simulink library "CH_Library"  (R2021a)
settings: Solver=VariableStepAuto  StartTime=0.0  StopTime=10.0  RelTol=1e-3
undefined symbols (not defined in the file or in its folder): Connection1, connection1, Connection2, connection2, Connection3, connection3, Connection4, connection4, Connection5, connection5, Connection6, connection6, Connection7, Connection8, FeetContact, HandContact, LeftArm, LeftFoot, params, RightArm, RightFoot, X, Y, Z
libraries: sm_lib x169, nesl_utility x40, $bdroot x16, sm_humanoid_walker_lib x13, fl_lib x10, simulink x7, ee_lib x3, simulink_extras x1
(part 2 of 5)

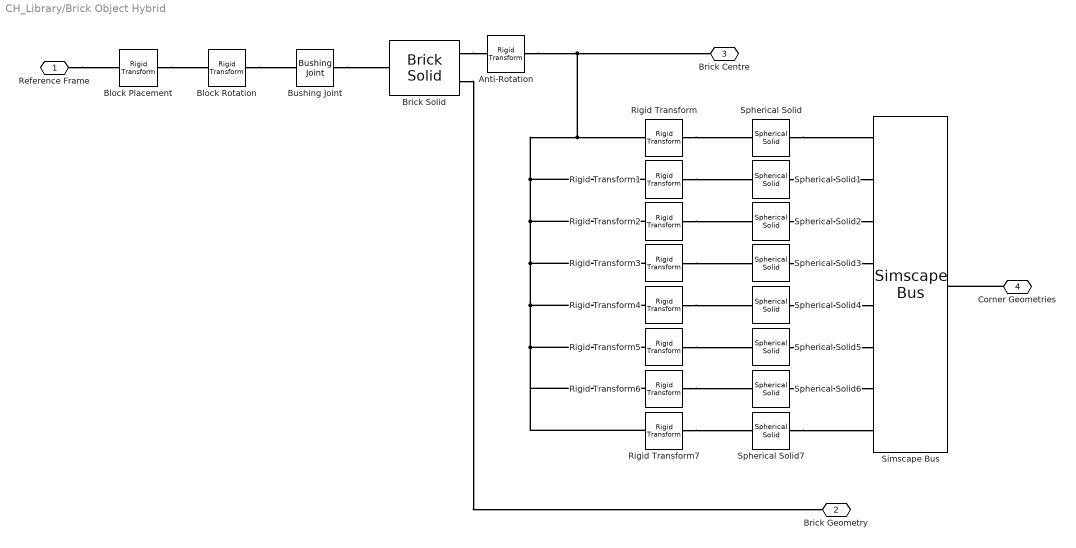
== system CH_Library/Brick Object Hybrid ==
  Anti-Rotation : sm_lib/Frames and Transforms/Rigid Transform  TranslationMethod=None  TranslationStandardOffset=0  TranslationLengthUnit=m  TranslationStandardAxis=+Z  TranslationCartesianOffset=[0 0 0]  TranslationROffset=0  TranslationROffsetUnits=m  TranslationZOffset=0  TranslationZOffsetUnits=m  TranslationThetaOffset=0  TranslationThetaOffsetUnits=deg  RotationMethod=RotationSequence  RotationAngleUnits=deg  RotationStandardAxis=+Z  RotationAngle=0.0  RotationArbitraryAxis=[0 0 1]  FollAlignAxisA=+X  BaseAlignAxisA=+Y  FollAlignAxisB=+Y  BaseAlignAxisB=+Z  RotationSequenceAxes=BaseAxes  RotationSequence=XYZ  RotationSequenceAngles=[-XRot -YRot -ZRot]  RotationSequenceAnglesUnits=deg  RotationMatrix=[1 0 0; 0 1 0; 0 0 1]
  Block Placement : sm_lib/Frames and Transforms/Rigid Transform  TranslationMethod=Cartesian  TranslationStandardOffset=0  TranslationLengthUnit=m  TranslationStandardAxis=+Z  TranslationCartesianOffset=[XDis YDis ZDis]  TranslationROffset=0  TranslationROffsetUnits=m  TranslationZOffset=0  TranslationZOffsetUnits=m  TranslationThetaOffset=0  TranslationThetaOffsetUnits=deg  RotationMethod=None  RotationAngleUnits=deg  RotationStandardAxis=+Z  RotationAngle=0.0  RotationArbitraryAxis=[0 0 1]  FollAlignAxisA=+X  BaseAlignAxisA=+Y  FollAlignAxisB=+Y  BaseAlignAxisB=+Z  RotationSequenceAxes=FollowerAxes  RotationSequence=XYX  RotationSequenceAngles=[0 0 0]  RotationSequenceAnglesUnits=deg  RotationMatrix=[1 0 0; 0 1 0; 0 0 1]
  Block Rotation : sm_lib/Frames and Transforms/Rigid Transform  TranslationMethod=None  TranslationStandardOffset=0  TranslationLengthUnit=m  TranslationStandardAxis=+Z  TranslationCartesianOffset=[0 0 0]  TranslationROffset=0  TranslationROffsetUnits=m  TranslationZOffset=0  TranslationZOffsetUnits=m  TranslationThetaOffset=0  TranslationThetaOffsetUnits=deg  RotationMethod=RotationSequence  RotationAngleUnits=deg  RotationStandardAxis=+Z  RotationAngle=0.0  RotationArbitraryAxis=[0 0 1]  FollAlignAxisA=+X  BaseAlignAxisA=+Y  FollAlignAxisB=+Y  BaseAlignAxisB=+Z  RotationSequenceAxes=BaseAxes  RotationSequence=XYZ  RotationSequenceAngles=[XRot YRot ZRot]  RotationSequenceAnglesUnits=deg  RotationMatrix=[1 0 0; 0 1 0; 0 0 1]
  Brick Solid : sm_lib/Body Elements/Brick Solid  GraphicAmbientColor=[0.15 0.15 0.15 1.0]  BasedOnType=Density  BrickDimensions=[BW BDep BH]  BrickDimensionUnits=m  CenterOfMass=[0 0 0]  CenterOfMassUnits=m  GraphicDiffuseColor=[BlockRed BlockGreen BlockBlue]  Density=BDen  DensityUnits=kg/m^3  DoExposeReferenceFrame=on  GraphicEmissiveColor=[0.0 0.0 0.0 1.0]  ExportEntireGeometry=on  SerializedFrames=<Frames><Frame><Id>Frame1</Id><Value><Name>Block Centre</Name><Origin><Source>ReferenceFrame</Source><FeatureName></FeatureName></Origin><PrimaryAxis><DefinedDirection>+Z</DefinedDirection><Source>ReferenceFrame</Source><SourceDirection>+Z</SourceDirection><FeatureName></FeatureName></PrimaryAxis><SecondaryAxis><DefinedDirection>+X</DefinedDirection><Source>ReferenceFrame</Source><SourceDirection>+X</SourceDirection><FeatureName></FeatureName></SecondaryAxis></Value></Frame></Frames>  MarkerShape=Sphere  MarkerSize=10  GraphicType=FromGeometry  InertiaType=CalculateFromGeometry  Mass=1  MassUnits=kg  MomentsOfInertia=[1 1 1]  MomentsOfInertiaUnits=kg*m^2  GraphicOpacity=BlockOpac  ProductsOfInertia=[0 0 0]  ProductsOfInertiaUnits=kg*m^2  GraphicShininess=75  GraphicSpecularColor=[0.5 0.5 0.5 1.0]  GraphicVisPropType=SimpleVisualProperties
  Bushing Joint : sm_lib/Joints/Bushing Joint  JointMode=Normal  SenseConstraintForce=off  SenseConstraintForceX=off  SenseConstraintForceY=off  SenseConstraintForceZ=off  SenseConstraintTorque=off  SenseConstraintTorqueX=off  SenseConstraintTorqueY=off  SenseConstraintTorqueZ=off  SenseTotalForce=off  SenseTotalForceX=off  SenseTotalForceY=off  SenseTotalForceZ=off  SenseTotalTorque=off  SenseTotalTorqueX=off  SenseTotalTorqueY=off  SenseTotalTorqueZ=off  CompositeWrenchDir=FollowerOnBase  CompositeWrenchFrame=BaseFrame  PxEquilibriumPosition=0  PxEquilibriumPositionUnits=m  PxSpringStiffness=0  PxSpringStiffnessUnits=N/m  PxDampingCoefficient=0  PxDampingCoefficientUnits=N/(m/s)  PxTorqueActuationMode=NoTorque  PxMotionActuationMode=ComputedMotion  PxSensePosition=off  PxSenseVelocity=off  PxSenseAcceleration=off  PxSenseTorqueForce=off  PxSenseLowerLimitTorqueForce=off  PxSenseUpperLimitTorqueForce=off  PxLowerLimitSpecify=off  PxLowerLimitBound=-1  PxLowerLimitBoundUnits=m  PxLowerLimitStiffness=1e6  PxLowerLimitStiffnessUnits=N/m  PxLowerLimitDamping=1e3  PxLowerLimitDampingUnits=N/(m/s)  PxLowerLimitTransitionRegionWidth=1e-4  PxLowerLimitTransitionRegionWidthUnits=m  PxUpperLimitSpecify=off  PxUpperLimitBound=1  PxUpperLimitBoundUnits=m  PxUpperLimitStiffness=1e6  PxUpperLimitStiffnessUnits=N/m  PxUpperLimitDamping=1e3  PxUpperLimitDampingUnits=N/(m/s)  PxUpperLimitTransitionRegionWidth=1e-4  PxUpperLimitTransitionRegionWidthUnits=m  PxPositionTargetSpecify=off  PxPositionTargetPriority=High  PxPositionTargetValue=0  PxPositionTargetValueUnits=m  PxVelocityTargetSpecify=off  PxVelocityTargetPriority=High  PxVelocityTargetValue=0  PxVelocityTargetValueUnits=m/s  PyEquilibriumPosition=0  PyEquilibriumPositionUnits=m  PySpringStiffness=0  PySpringStiffnessUnits=N/m  PyDampingCoefficient=0  PyDampingCoefficientUnits=N/(m/s)  PyTorqueActuationMode=NoTorque  PyMotionActuationMode=ComputedMotion  PySensePosition=off  PySenseVelocity=off  PySenseAcceleration=off  PySenseTorqueForce=off  PySenseLowerLimitTorqueForce=off  PySenseUpperLimitTorqueForce=off  PyLowerLimitSpecify=off  PyLowerLimitBound=-1  PyLowerLimitBoundUnits=m  PyLowerLimitStiffness=1e6  PyLowerLimitStiffnessUnits=N/m  PyLowerLimitDamping=1e3  PyLowerLimitDampingUnits=N/(m/s)  PyLowerLimitTransitionRegionWidth=1e-4  PyLowerLimitTransitionRegionWidthUnits=m  PyUpperLimitSpecify=off  PyUpperLimitBound=1  PyUpperLimitBoundUnits=m  PyUpperLimitStiffness=1e6  PyUpperLimitStiffnessUnits=N/m  PyUpperLimitDamping=1e3  PyUpperLimitDampingUnits=N/(m/s)  PyUpperLimitTransitionRegionWidth=1e-4  PyUpperLimitTransitionRegionWidthUnits=m  PyPositionTargetSpecify=off  PyPositionTargetPriority=High  PyPositionTargetValue=0  PyPositionTargetValueUnits=m  PyVelocityTargetSpecify=off  PyVelocityTargetPriority=High  PyVelocityTargetValue=0  PyVelocityTargetValueUnits=m/s  PzEquilibriumPosition=0  PzEquilibriumPositionUnits=m  PzSpringStiffness=0  PzSpringStiffnessUnits=N/m  PzDampingCoefficient=0  PzDampingCoefficientUnits=N/(m/s)  PzTorqueActuationMode=NoTorque  PzMotionActuationMode=ComputedMotion  PzSensePosition=off  PzSenseVelocity=off  PzSenseAcceleration=off  PzSenseTorqueForce=off  PzSenseLowerLimitTorqueForce=off  PzSenseUpperLimitTorqueForce=off  PzLowerLimitSpecify=off  PzLowerLimitBound=-1  PzLowerLimitBoundUnits=m  PzLowerLimitStiffness=1e6  PzLowerLimitStiffnessUnits=N/m  PzLowerLimitDamping=1e3  PzLowerLimitDampingUnits=N/(m/s)  PzLowerLimitTransitionRegionWidth=1e-4  PzLowerLimitTransitionRegionWidthUnits=m  PzUpperLimitSpecify=off  PzUpperLimitBound=1  PzUpperLimitBoundUnits=m  PzUpperLimitStiffness=1e6  PzUpperLimitStiffnessUnits=N/m  PzUpperLimitDamping=1e3  PzUpperLimitDampingUnits=N/(m/s)  PzUpperLimitTransitionRegionWidth=1e-4  PzUpperLimitTransitionRegionWidthUnits=m  PzPositionTargetSpecify=off  PzPositionTargetPriority=High  PzPositionTargetValue=0  PzPositionTargetValueUnits=m  PzVelocityTargetSpecify=off  PzVelocityTargetPriority=High  PzVelocityTargetValue=0  PzVelocityTargetValueUnits=m/s  RxEquilibriumPosition=0  RxEquilibriumPositionUnits=deg  RxSpringStiffness=0  RxSpringStiffnessUnits=N*m/deg  RxDampingCoefficient=0  RxDampingCoefficientUnits=N*m/(deg/s)  RxTorqueActuationMode=NoTorque  RxMotionActuationMode=ComputedMotion  RxSensePosition=off  RxSenseVelocity=off  RxSenseAcceleration=off  RxSenseTorqueForce=off  RxSenseLowerLimitTorqueForce=off  RxSenseUpperLimitTorqueForce=off  RxLowerLimitSpecify=off  RxLowerLimitBound=-90  RxLowerLimitBoundUnits=deg  RxLowerLimitStiffness=1e4  RxLowerLimitStiffnessUnits=N*m/deg  RxLowerLimitDamping=10  RxLowerLimitDampingUnits=N*m/(deg/s)  RxLowerLimitTransitionRegionWidth=0.1  RxLowerLimitTransitionRegionWidthUnits=deg  RxUpperLimitSpecify=off  RxUpperLimitBound=90  RxUpperLimitBoundUnits=deg  RxUpperLimitStiffness=1e4  RxUpperLimitStiffnessUnits=N*m/deg  RxUpperLimitDamping=10  RxUpperLimitDampingUnits=N*m/(deg/s)  RxUpperLimitTransitionRegionWidth=0.1  RxUpperLimitTransitionRegionWidthUnits=deg  RxPositionTargetSpecify=off  RxPositionTargetPriority=High  RxPositionTargetValue=0  RxPositionTargetValueUnits=deg  RxVelocityTargetSpecify=off  RxVelocityTargetPriority=High  RxVelocityTargetValue=0  RxVelocityTargetValueUnits=deg/s  RyEquilibriumPosition=0  RyEquilibriumPositionUnits=deg  RySpringStiffness=0  RySpringStiffnessUnits=N*m/deg  RyDampingCoefficient=0  RyDampingCoefficientUnits=N*m/(deg/s)  RyTorqueActuationMode=NoTorque  RyMotionActuationMode=ComputedMotion  RySensePosition=off  RySenseVelocity=off  RySenseAcceleration=off  RySenseTorqueForce=off  RySenseLowerLimitTorqueForce=off  RySenseUpperLimitTorqueForce=off  RyLowerLimitSpecify=off  RyLowerLimitBound=-90  RyLowerLimitBoundUnits=deg  RyLowerLimitStiffness=1e4  RyLowerLimitStiffnessUnits=N*m/deg  RyLowerLimitDamping=10  RyLowerLimitDampingUnits=N*m/(deg/s)  RyLowerLimitTransitionRegionWidth=0.1  RyLowerLimitTransitionRegionWidthUnits=deg  RyUpperLimitSpecify=off  RyUpperLimitBound=90  RyUpperLimitBoundUnits=deg  RyUpperLimitStiffness=1e4  RyUpperLimitStiffnessUnits=N*m/deg  RyUpperLimitDamping=10  RyUpperLimitDampingUnits=N*m/(deg/s)  RyUpperLimitTransitionRegionWidth=0.1  RyUpperLimitTransitionRegionWidthUnits=deg  RyPositionTargetSpecify=off  RyPositionTargetPriority=High  RyPositionTargetValue=0  RyPositionTargetValueUnits=deg  RyVelocityTargetSpecify=off  RyVelocityTargetPriority=High  RyVelocityTargetValue=0  RyVelocityTargetValueUnits=deg/s  RzEquilibriumPosition=0  RzEquilibriumPositionUnits=deg  RzSpringStiffness=0  RzSpringStiffnessUnits=N*m/deg  RzDampingCoefficient=0  RzDampingCoefficientUnits=N*m/(deg/s)  RzTorqueActuationMode=NoTorque  RzMotionActuationMode=ComputedMotion  RzSensePosition=off  RzSenseVelocity=off  RzSenseAcceleration=off  RzSenseTorqueForce=off  RzSenseLowerLimitTorqueForce=off  RzSenseUpperLimitTorqueForce=off  RzLowerLimitSpecify=off  RzLowerLimitBound=-90  RzLowerLimitBoundUnits=deg  RzLowerLimitStiffness=1e4  RzLowerLimitStiffnessUnits=N*m/deg  RzLowerLimitDamping=10  RzLowerLimitDampingUnits=N*m/(deg/s)  RzLowerLimitTransitionRegionWidth=0.1  RzLowerLimitTransitionRegionWidthUnits=deg  RzUpperLimitSpecify=off  RzUpperLimitBound=90  RzUpperLimitBoundUnits=deg  RzUpperLimitStiffness=1e4  RzUpperLimitStiffnessUnits=N*m/deg  RzUpperLimitDamping=10  RzUpperLimitDampingUnits=N*m/(deg/s)  RzUpperLimitTransitionRegionWidth=0.1  RzUpperLimitTransitionRegionWidthUnits=deg  RzPositionTargetSpecify=off  RzPositionTargetPriority=High  RzPositionTargetValue=0  RzPositionTargetValueUnits=deg  RzVelocityTargetSpecify=off  RzVelocityTargetPriority=High  RzVelocityTargetValue=0  RzVelocityTargetValueUnits=deg/s
  Rigid Transform : sm_lib/Frames and Transforms/Rigid Transform  TranslationMethod=Cartesian  TranslationStandardOffset=0  TranslationLengthUnit=m  TranslationStandardAxis=+Z  TranslationCartesianOffset=[BW BH BDep]/2  TranslationROffset=0  TranslationROffsetUnits=m  TranslationZOffset=0  TranslationZOffsetUnits=m  TranslationThetaOffset=0  TranslationThetaOffsetUnits=deg  RotationMethod=None  RotationAngleUnits=deg  RotationStandardAxis=+Z  RotationAngle=0.0  RotationArbitraryAxis=[0 0 1]  FollAlignAxisA=+X  BaseAlignAxisA=+Y  FollAlignAxisB=+Y  BaseAlignAxisB=+Z  RotationSequenceAxes=FollowerAxes  RotationSequence=XYX  RotationSequenceAngles=[0 0 0]  RotationSequenceAnglesUnits=deg  RotationMatrix=[1 0 0; 0 1 0; 0 0 1]
  Rigid Transform1 : sm_lib/Frames and Transforms/Rigid Transform  TranslationMethod=Cartesian  TranslationStandardOffset=0  TranslationLengthUnit=m  TranslationStandardAxis=+Z  TranslationCartesianOffset=[BW BH -BDep]/2  TranslationROffset=0  TranslationROffsetUnits=m  TranslationZOffset=0  TranslationZOffsetUnits=m  TranslationThetaOffset=0  TranslationThetaOffsetUnits=deg  RotationMethod=None  RotationAngleUnits=deg  RotationStandardAxis=+Z  RotationAngle=0.0  RotationArbitraryAxis=[0 0 1]  FollAlignAxisA=+X  BaseAlignAxisA=+Y  FollAlignAxisB=+Y  BaseAlignAxisB=+Z  RotationSequenceAxes=FollowerAxes  RotationSequence=XYX  RotationSequenceAngles=[0 0 0]  RotationSequenceAnglesUnits=deg  RotationMatrix=[1 0 0; 0 1 0; 0 0 1]
  Rigid Transform2 : sm_lib/Frames and Transforms/Rigid Transform  TranslationMethod=Cartesian  TranslationStandardOffset=0  TranslationLengthUnit=m  TranslationStandardAxis=+Z  TranslationCartesianOffset=[BW -BH BDep]/2  TranslationROffset=0  TranslationROffsetUnits=m  TranslationZOffset=0  TranslationZOffsetUnits=m  TranslationThetaOffset=0  TranslationThetaOffsetUnits=deg  RotationMethod=None  RotationAngleUnits=deg  RotationStandardAxis=+Z  RotationAngle=0.0  RotationArbitraryAxis=[0 0 1]  FollAlignAxisA=+X  BaseAlignAxisA=+Y  FollAlignAxisB=+Y  BaseAlignAxisB=+Z  RotationSequenceAxes=FollowerAxes  RotationSequence=XYX  RotationSequenceAngles=[0 0 0]  RotationSequenceAnglesUnits=deg  RotationMatrix=[1 0 0; 0 1 0; 0 0 1]
  Rigid Transform3 : sm_lib/Frames and Transforms/Rigid Transform  TranslationMethod=Cartesian  TranslationStandardOffset=0  TranslationLengthUnit=m  TranslationStandardAxis=+Z  TranslationCartesianOffset=[BW -BH -BDep]/2  TranslationROffset=0  TranslationROffsetUnits=m  TranslationZOffset=0  TranslationZOffsetUnits=m  TranslationThetaOffset=0  TranslationThetaOffsetUnits=deg  RotationMethod=None  RotationAngleUnits=deg  RotationStandardAxis=+Z  RotationAngle=0.0  RotationArbitraryAxis=[0 0 1]  FollAlignAxisA=+X  BaseAlignAxisA=+Y  FollAlignAxisB=+Y  BaseAlignAxisB=+Z  RotationSequenceAxes=FollowerAxes  RotationSequence=XYX  RotationSequenceAngles=[0 0 0]  RotationSequenceAnglesUnits=deg  RotationMatrix=[1 0 0; 0 1 0; 0 0 1]
  Rigid Transform4 : sm_lib/Frames and Transforms/Rigid Transform  TranslationMethod=Cartesian  TranslationStandardOffset=0  TranslationLengthUnit=m  TranslationStandardAxis=+Z  TranslationCartesianOffset=[-BW BH BDep]/2  TranslationROffset=0  TranslationROffsetUnits=m  TranslationZOffset=0  TranslationZOffsetUnits=m  TranslationThetaOffset=0  TranslationThetaOffsetUnits=deg  RotationMethod=None  RotationAngleUnits=deg  RotationStandardAxis=+Z  RotationAngle=0.0  RotationArbitraryAxis=[0 0 1]  FollAlignAxisA=+X  BaseAlignAxisA=+Y  FollAlignAxisB=+Y  BaseAlignAxisB=+Z  RotationSequenceAxes=FollowerAxes  RotationSequence=XYX  RotationSequenceAngles=[0 0 0]  RotationSequenceAnglesUnits=deg  RotationMatrix=[1 0 0; 0 1 0; 0 0 1]
  Rigid Transform5 : sm_lib/Frames and Transforms/Rigid Transform  TranslationMethod=Cartesian  TranslationStandardOffset=0  TranslationLengthUnit=m  TranslationStandardAxis=+Z  TranslationCartesianOffset=[-BW BH -BDep]/2  TranslationROffset=0  TranslationROffsetUnits=m  TranslationZOffset=0  TranslationZOffsetUnits=m  TranslationThetaOffset=0  TranslationThetaOffsetUnits=deg  RotationMethod=None  RotationAngleUnits=deg  RotationStandardAxis=+Z  RotationAngle=0.0  RotationArbitraryAxis=[0 0 1]  FollAlignAxisA=+X  BaseAlignAxisA=+Y  FollAlignAxisB=+Y  BaseAlignAxisB=+Z  RotationSequenceAxes=FollowerAxes  RotationSequence=XYX  RotationSequenceAngles=[0 0 0]  RotationSequenceAnglesUnits=deg  RotationMatrix=[1 0 0; 0 1 0; 0 0 1]
  Rigid Transform6 : sm_lib/Frames and Transforms/Rigid Transform  TranslationMethod=Cartesian  TranslationStandardOffset=0  TranslationLengthUnit=m  TranslationStandardAxis=+Z  TranslationCartesianOffset=[-BW -BH BDep]/2  TranslationROffset=0  TranslationROffsetUnits=m  TranslationZOffset=0  TranslationZOffsetUnits=m  TranslationThetaOffset=0  TranslationThetaOffsetUnits=deg  RotationMethod=None  RotationAngleUnits=deg  RotationStandardAxis=+Z  RotationAngle=0.0  RotationArbitraryAxis=[0 0 1]  FollAlignAxisA=+X  BaseAlignAxisA=+Y  FollAlignAxisB=+Y  BaseAlignAxisB=+Z  RotationSequenceAxes=FollowerAxes  RotationSequence=XYX  RotationSequenceAngles=[0 0 0]  RotationSequenceAnglesUnits=deg  RotationMatrix=[1 0 0; 0 1 0; 0 0 1]
  Rigid Transform7 : sm_lib/Frames and Transforms/Rigid Transform  TranslationMethod=Cartesian  TranslationStandardOffset=0  TranslationLengthUnit=m  TranslationStandardAxis=+Z  TranslationCartesianOffset=[-BW -BH -BDep]/2  TranslationROffset=0  TranslationROffsetUnits=m  TranslationZOffset=0  TranslationZOffsetUnits=m  TranslationThetaOffset=0  TranslationThetaOffsetUnits=deg  RotationMethod=None  RotationAngleUnits=deg  RotationStandardAxis=+Z  RotationAngle=0.0  RotationArbitraryAxis=[0 0 1]  FollAlignAxisA=+X  BaseAlignAxisA=+Y  FollAlignAxisB=+Y  BaseAlignAxisB=+Z  RotationSequenceAxes=FollowerAxes  RotationSequence=XYX  RotationSequenceAngles=[0 0 0]  RotationSequenceAnglesUnits=deg  RotationMatrix=[1 0 0; 0 1 0; 0 0 1]
  Simscape Bus : SimscapeBus  HierarchyStrings=Connection1;Connection2;Connection3;Connection4;Connection5;Connection6;Connection7;Connection8
  Spherical Solid{,1..7} (8 alike) : sm_lib/Body Elements/Spherical Solid  GraphicAmbientColor=[0.15 0.15 0.15 1.0]  BasedOnType=Density  CenterOfMass=[0 0 0]  CenterOfMassUnits=m  GraphicDiffuseColor=[0.5 0.5 0.5]  Density=0.01  DensityUnits=kg/m^3  DoExposeReferenceFrame=on  GraphicEmissiveColor=[0.0 0.0 0.0 1.0]  ExportEntireGeometry=on  SerializedExposedGeometries=<ExposedGeometries><ExposedGeometry><RawGeometryId>entire</RawGeometryId><ExposedGeometryId>G</ExposedGeometryId></ExposedGeometry></ExposedGeometries>  SerializedFrames=<Frames/>  MarkerShape=Sphere  MarkerSize=10  GraphicType=FromGeometry  InertiaType=CalculateFromGeometry  Mass=1  MassUnits=kg  MomentsOfInertia=[1 1 1]  MomentsOfInertiaUnits=kg*m^2  GraphicOpacity=0  ProductsOfInertia=[0 0 0]  ProductsOfInertiaUnits=kg*m^2  GraphicShininess=75  GraphicSpecularColor=[0.5 0.5 0.5 1.0]  SphereRadius=0.1  SphereRadiusUnits=m  GraphicVisPropType=SimpleVisualProperties
  Reference Frame : PMIOPort  Side=Left
  Brick Geometry : PMIOPort  Port=2  Side=Right
  Brick Centre : PMIOPort  Port=3  Side=Right
  Corner Geometries : PMIOPort  Port=4  Side=Right
  connections:
  Bushing Joint/RConn1 -- Brick Solid/RConn1
  Reference Frame/RConn1 -- Block Placement/LConn1
  Block Placement/RConn1 -- Block Rotation/LConn1
  Block Rotation/RConn1 -- Bushing Joint/LConn1
  Brick Solid/LConn1 -- Anti-Rotation/LConn1
  Rigid Transform3/LConn1 -- Rigid Transform/LConn1 -- Brick Centre/RConn1 -- Anti-Rotation/RConn1 -- Rigid Transform1/LConn1 -- Rigid Transform2/LConn1 -- Rigid Transform4/LConn1 -- Rigid Transform5/LConn1 -- Rigid Transform6/LConn1 -- Rigid Transform7/LConn1
  Brick Solid/LConn2 -- Brick Geometry/RConn1
  Spherical Solid4/LConn1 -- Simscape Bus/LConn5
  Rigid Transform6/RConn1 -- Spherical Solid6/RConn1
  Spherical Solid6/LConn1 -- Simscape Bus/LConn7
  Spherical Solid2/LConn1 -- Simscape Bus/LConn3
  Spherical Solid1/LConn1 -- Simscape Bus/LConn2
  Spherical Solid/LConn1 -- Simscape Bus/LConn1
  Spherical Solid3/LConn1 -- Simscape Bus/LConn4
  Rigid Transform5/RConn1 -- Spherical Solid5/RConn1
  Rigid Transform/RConn1 -- Spherical Solid/RConn1
  Rigid Transform1/RConn1 -- Spherical Solid1/RConn1
  Rigid Transform4/RConn1 -- Spherical Solid4/RConn1
  Spherical Solid7/LConn1 -- Simscape Bus/LConn8
  Spherical Solid5/LConn1 -- Simscape Bus/LConn6
  Rigid Transform7/RConn1 -- Spherical Solid7/RConn1
  Rigid Transform2/RConn1 -- Spherical Solid2/RConn1
  Corner Geometries/RConn1 -- Simscape Bus/RConn1
  Rigid Transform3/RConn1 -- Spherical Solid3/RConn1

== system CH_Library/Calculate Power ==
  Joint Sensing : Inport
  Joint Torques : Inport  Port=2
  Bus Selector1 : BusSelector  OutputSignals=LegSense.RightLegSense.RHS.rhThetaDot,LegSense.RightLegSense.RKS.rkThetaDot,LegSense.RightLegSense.RAS.raThetaDot,LegSense.LeftLegSense.LHS.lhThetaDot,LegSense.LeftLegSense.LKS.lkThetaDot,LegSense.LeftLegSense.LAS.laThetaDot,ArmSense.LeftArmSense.LWS.lwThetaDot,ArmSense.LeftArmSense.LES.leThetaDot,ArmSense.LeftArmSense.LSSS.lssThetaDot,ArmSense.LeftArmSense.LSFS.lsfThetaDot,ArmSense.RightArmSense.RWS.rwThetaDot,ArmSense.RightArmSense.RES.reThetaDot,ArmSense.RightArmSense.RSSS.rssThetaDot,ArmSense.RightArmSense.RSFS.rsfThetaDot
  Mux : Mux  Inputs=14
  Product : Product
  Sum of Elements : Sum  Inputs=+
  Unit Delay : UnitDelay  SampleTime=-1  HasFrameUpgradeWarning=on
  Total Power : Outport
  wires:
  Bus Selector1/7 -> Mux/7  "<lwThetaDot>"
  Bus Selector1/8 -> Mux/8  "<leThetaDot>"
  Bus Selector1/9 -> Mux/9  "<lssThetaDot>"
  Bus Selector1/10 -> Mux/10  "<lsfThetaDot>"
  Bus Selector1/11 -> Mux/11  "<rwThetaDot>"
  Bus Selector1/12 -> Mux/12  "<reThetaDot>"
  Bus Selector1/13 -> Mux/13  "<rssThetaDot>"
  Bus Selector1/14 -> Mux/14  "<rsfThetaDot>"
  Product/1 -> Sum of Elements/1
  Joint Sensing/1 -> Bus Selector1/1
  Mux/1 -> Product/1
  Joint Torques/1 -> Product/2
  Sum of Elements/1 -> Unit Delay/1
  Bus Selector1/1 -> Mux/1  "<rhThetaDot>"
  Bus Selector1/2 -> Mux/2  "<rkThetaDot>"
  Bus Selector1/3 -> Mux/3  "<raThetaDot>"
  Bus Selector1/4 -> Mux/4  "<lhThetaDot>"
  Bus Selector1/5 -> Mux/5  "<lkThetaDot>"
  Bus Selector1/6 -> Mux/6  "<laThetaDot>"
  Unit Delay/1 -> Total Power/1

== system CH_Library/Calculate Reward ==
  Torso Sensing : Inport
  Power : Inport  Port=2
  Box Motion : Inport  Port=3
  " " : Gain  Gain=-lateralPenalty
  "     " : Gain  Gain=-verticalPenalty
  "                    " : Gain  Gain=-powerPenalty
  "                       " : Constant  Value=timestepReward*params.simulation.Ts
  "                    1" : Gain  Gain=BoxReward
  Bus Creator : BusCreator  Inputs=6
  Bus Selector : BusSelector  OutputSignals=signal2.vrad,signal2.x,signal2.dz
  Gain : Gain  Gain=forwardReward
  Rate Transition2 : RateTransition  OutPortSampleTime=params.simulation.Ts
  Square3 : Math  Operator=square  SignedPower=on  SaturateOnIntegerOverflow=on
  Square4 : Math  Operator=square  SignedPower=on  SaturateOnIntegerOverflow=on
  Sum of Elements : Sum  Inputs=+
  Reward : Outport  VectorParamsAs1DForOutWhenUnconnected=off
  Reward Components : Outport  Port=2  VectorParamsAs1DForOutWhenUnconnected=off
  wires:
  Torso Sensing/1 -> Bus Selector/1
  Power/1 -> "                    "/1
  Square4/1 -> "     "/1
  Bus Selector/3 -> Square4/1  "<dz>"
  Square3/1 -> " "/1
  Bus Selector/2 -> Square3/1  "<x>"
  Sum of Elements/1 -> Reward/1
  " "/1 -> Bus Creator/3  "Lateral Penalty"
  "                    "/1 -> Bus Creator/5  "Power Penalty"
  "                       "/1 -> Bus Creator/1  "Duration Reward"
  Bus Selector/1 -> Gain/1  "<vrad>"
  Gain/1 -> Bus Creator/2  "Forward Reward"
  "     "/1 -> Bus Creator/4  "Vertical Penalty"
  Bus Creator/1 -> Rate Transition2/1
  Rate Transition2/1 -> Reward Components/1, Sum of Elements/1
  Box Motion/1 -> "                    1"/1
  "                    1"/1 -> Bus Creator/6  "Box Motion Reward"

== system CH_Library/Camera ==
  Camera Location : sm_lib/Frames and Transforms/Rigid Transform  TranslationMethod=Cartesian  TranslationStandardOffset=0  TranslationLengthUnit=m  TranslationStandardAxis=+Z  TranslationCartesianOffset=[X_TF Y_TF Z_TF]  TranslationROffset=0  TranslationROffsetUnits=m  TranslationZOffset=0  TranslationZOffsetUnits=m  TranslationThetaOffset=0  TranslationThetaOffsetUnits=deg  RotationMethod=None  RotationAngleUnits=deg  RotationStandardAxis=+Z  RotationAngle=0.0  RotationArbitraryAxis=[0 0 1]  FollAlignAxisA=+X  BaseAlignAxisA=+Y  FollAlignAxisB=+Y  BaseAlignAxisB=+Z  RotationSequenceAxes=FollowerAxes  RotationSequence=XYX  RotationSequenceAngles=[0 0 0]  RotationSequenceAnglesUnits=deg  RotationMatrix=[1 0 0; 0 1 0; 0 0 1]
  Camera Rotation : sm_lib/Frames and Transforms/Rigid Transform  TranslationMethod=None  TranslationStandardOffset=0  TranslationLengthUnit=m  TranslationStandardAxis=+Z  TranslationCartesianOffset=[0 0 0]  TranslationROffset=0  TranslationROffsetUnits=m  TranslationZOffset=0  TranslationZOffsetUnits=m  TranslationThetaOffset=0  TranslationThetaOffsetUnits=deg  RotationMethod=RotationSequence  RotationAngleUnits=deg  RotationStandardAxis=+Z  RotationAngle=0.0  RotationArbitraryAxis=[0 0 1]  FollAlignAxisA=+X  BaseAlignAxisA=+Y  FollAlignAxisB=+Y  BaseAlignAxisB=+Z  RotationSequenceAxes=FollowerAxes  RotationSequence=ZXZ  RotationSequenceAngles=[Z_ROT X_ROT 0]  RotationSequenceAnglesUnits=deg  RotationMatrix=[1 0 0; 0 1 0; 0 0 1]
  Spherical Solid : sm_lib/Body Elements/Spherical Solid  GraphicAmbientColor=[0.15 0.15 0.15 1.0]  BasedOnType=Density  CenterOfMass=[0 0 0]  CenterOfMassUnits=m  GraphicDiffuseColor=[0.2 1.0 0.2]  Density=1000  DensityUnits=kg/m^3  DoExposeReferenceFrame=on  GraphicEmissiveColor=[0.0 0.0 0.0 1.0]  ExportEntireGeometry=off  SerializedExposedGeometries=<ExposedGeometries/>  SerializedFrames=<Frames/>  MarkerShape=Sphere  MarkerSize=10  GraphicType=FromGeometry  InertiaType=PointMass  Mass=1  MassUnits=g  MomentsOfInertia=[1 1 1]  MomentsOfInertiaUnits=kg*m^2  GraphicOpacity=1.0  ProductsOfInertia=[0 0 0]  ProductsOfInertiaUnits=kg*m^2  GraphicShininess=75  GraphicSpecularColor=[0.5 0.5 0.5 1.0]  SphereRadius=0.01  SphereRadiusUnits=m  GraphicVisPropType=SimpleVisualProperties
  Camera : PMIOPort  Side=Right
  connections:
  Spherical Solid/RConn1 -- Camera Location/RConn1
  Camera Rotation/RConn1 -- Camera Location/LConn1
  Camera/RConn1 -- Camera Rotation/LConn1

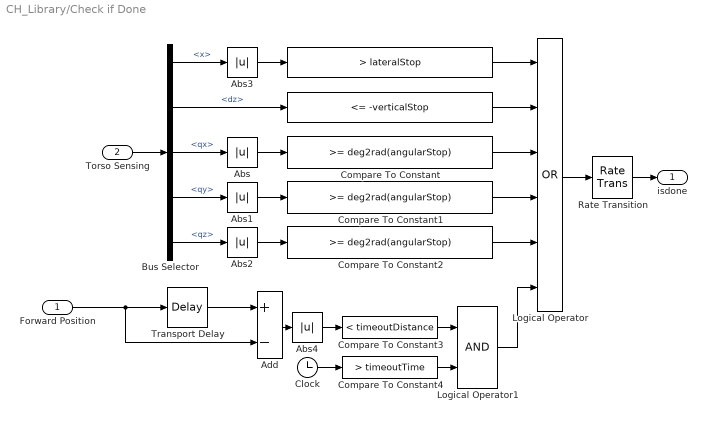
== system CH_Library/Check if Done ==
  Forward Position : Inport
  Torso Sensing : Inport  Port=2
  " " : simulink/Logic and Bit Operations/Compare To Constant  relop=<=  const=-verticalStop  OutDataTypeStr=boolean  ZeroCross=off
  "             " : simulink/Logic and Bit Operations/Compare To Constant  relop=>  const=lateralStop  OutDataTypeStr=boolean
  Abs{,1..3} (4 alike) : Abs  ZeroCross=off
  Abs4 : Abs
  Add : Sum  Inputs=+-
  Bus Selector : BusSelector  OutputSignals=signal2.x,signal2.dz,signal1.qx,signal1.qy,signal1.qz
  Clock : Clock
  Compare To Constant : simulink/Logic and Bit Operations/Compare To Constant  relop=>=  const=deg2rad(angularStop)  OutDataTypeStr=boolean  ZeroCross=off
  Compare To Constant1 : simulink/Logic and Bit Operations/Compare To Constant  relop=>=  const=deg2rad(angularStop)  OutDataTypeStr=boolean  ZeroCross=off
  Compare To Constant2 : simulink/Logic and Bit Operations/Compare To Constant  relop=>=  const=deg2rad(angularStop)  OutDataTypeStr=boolean  ZeroCross=off
  Compare To Constant3 : simulink/Logic and Bit Operations/Compare To Constant  relop=<  const=timeoutDistance  OutDataTypeStr=boolean
  Compare To Constant4 : simulink/Logic and Bit Operations/Compare To Constant  relop=>  const=timeoutTime  OutDataTypeStr=boolean
  Logical Operator : Logic  Operator=OR  Inputs=6  AllPortsSameDT=off  OutDataTypeStr=boolean
  Logical Operator1 : Logic  AllPortsSameDT=off  OutDataTypeStr=boolean
  Rate Transition : RateTransition  OutPortSampleTime=params.simulation.Ts
  Transport Delay : TransportDelay  DelayTime=timeoutTime  BufferSize=8192
  isdone : Outport  VectorParamsAs1DForOutWhenUnconnected=off
  wires:
  Bus Selector/2 -> " "/1  "<dz>"
  Torso Sensing/1 -> Bus Selector/1
  " "/1 -> Logical Operator/2
  Bus Selector/3 -> Abs/1  "<qx>"
  Bus Selector/4 -> Abs1/1  "<qy>"
  Compare To Constant/1 -> Logical Operator/3
  Abs/1 -> Compare To Constant/1
  Abs1/1 -> Compare To Constant1/1
  Logical Operator/1 -> Rate Transition/1
  Abs3/1 -> "             "/1
  Bus Selector/1 -> Abs3/1  "<x>"
  "             "/1 -> Logical Operator/1
  Abs2/1 -> Compare To Constant2/1
  Bus Selector/5 -> Abs2/1  "<qz>"
  Compare To Constant2/1 -> Logical Operator/5
  Compare To Constant1/1 -> Logical Operator/4
  Rate Transition/1 -> isdone/1
  Forward Position/1 -> Add/2, Transport Delay/1
  Transport Delay/1 -> Add/1
  Add/1 -> Abs4/1
  Abs4/1 -> Compare To Constant3/1
  Clock/1 -> Compare To Constant4/1
  Logical Operator1/1 -> Logical Operator/6
  Compare To Constant3/1 -> Logical Operator1/1
  Compare To Constant4/1 -> Logical Operator1/2

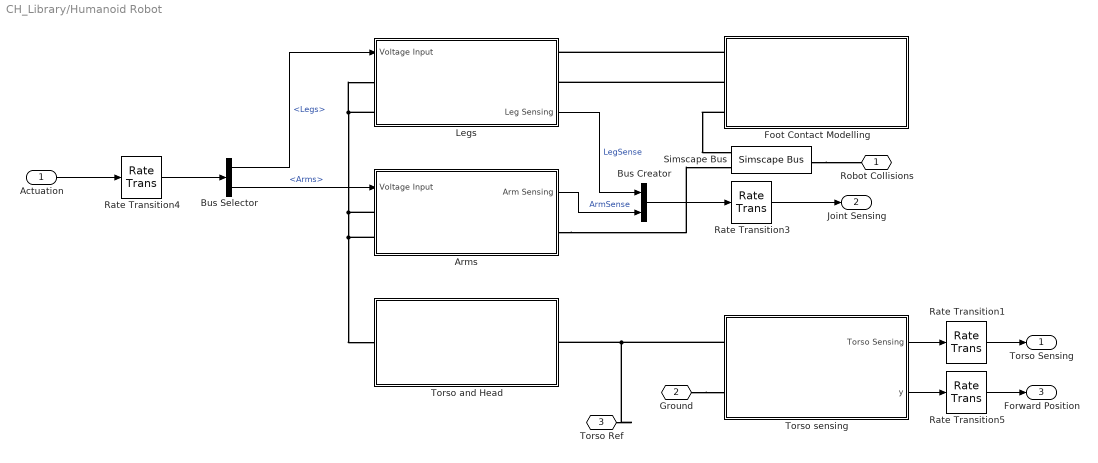
== system CH_Library/Humanoid Robot ==
  Actuation : Inport
  Arms : Subsystem
  Bus Creator : BusCreator  Inputs=2
  Bus Selector : BusSelector  OutputSignals=Legs,Arms
  Foot Contact Modelling : Subsystem
  Legs : Subsystem
      settings: PortSchema="{\"entries\":[{\"content\":{\"sides\":[{\"content\":{\"connectorIds\":[\"In1\",\"LConn1\",\"LConn2\"]},\"type\":\"ConnectorPlacement.EquallySpacedRectSide\",\"uuid\":\"23351413-746b-4a06-be1b-12a3513cfbfe\"},{\"content\":{\"connectorIds\":[\"RConn1\",\"RConn2\",\"Out1\"],\"side\":\"RIGHT\"},\"type\":\"ConnectorPlacement.EquallySpacedRectSide\",\"uuid\":\"11cf50da-2174-4e1a-8294-03a32c066ee9\"},{\"content\":{\"connectorIds\":[],\"side\":\"TOP\"},\"type\":\"ConnectorPlacement.EquallySpacedRectSide\",\"uuid\":\"131464a5-eb41-49e4-a10b-6e29adf56ddb\"}]},\"type\":\"ConnectorPlacement.EquallySpacedConnector\",\"uuid\":\"d1829b9e-a701-4b79-9220-5146acc6850e\"}],\"packageUris\":[\"http://schema.mathworks.com/mf0/Connector/R2020b\"],\"version\":\"1.0\"}"
  Rate Transition{1,3..5} (4 alike) : RateTransition  OutPortSampleTime=params.simulation.Ts
  Simscape Bus : SimscapeBus  HierarchyStrings=FeetContact;HandContact
  Torso and Head : Subsystem
  Torso sensing : Subsystem
  Robot Collisions : PMIOPort  Side=Right
  " Ground" : PMIOPort  Port=2  Side=Left
  Torso Ref : PMIOPort  Port=3  Side=Left
  Torso Sensing : Outport
  Joint Sensing : Outport  Port=2
  Forward Position : Outport  Port=3
  wires:
  Actuation/1 -> Rate Transition4/1
  Torso sensing/1(Torso Sensing) -> Rate Transition1/1
  Rate Transition1/1 -> Torso Sensing/1
  Rate Transition3/1 -> Joint Sensing/1
  Rate Transition5/1 -> Forward Position/1
  Torso sensing/2(y) -> Rate Transition5/1
  Rate Transition4/1 -> Bus Selector/1
  Bus Selector/1 -> Legs/1(Voltage Input)  "<Legs>"
  Bus Selector/2 -> Arms/1(Voltage Input)  "<Arms>"
  Bus Creator/1 -> Rate Transition3/1
  Legs/1(Leg Sensing) -> Bus Creator/1  "LegSense"
  Arms/1(Arm Sensing) -> Bus Creator/2  "ArmSense"
  connections:
  Legs/LConn2 -- Legs/LConn1 -- Arms/LConn1 -- Arms/LConn2 -- Torso and Head/LConn1
  Torso sensing/LConn1 -- Torso Ref/RConn1 -- Torso and Head/RConn1
  Foot Contact Modelling/LConn1 -- Legs/RConn1
  Foot Contact Modelling/LConn2 -- Legs/RConn2
  " Ground"/RConn1 -- Torso sensing/LConn2
  Foot Contact Modelling/LConn3 -- Simscape Bus/LConn1
  Arms/RConn1 -- Simscape Bus/LConn2
  Simscape Bus/RConn1 -- Robot Collisions/RConn1

== system CH_Library/Joint Controller ==
  Control Input : Inport
  Joint Position : Inport  Port=2
  Joint Velocity : Inport  Port=3
  Add Constant : Bias  Bias=jointLowerLimit + (jointUpperLimit-jointLowerLimit)/2
  Damping : Gain  Gain=jointDamping
  Degrees to Radians : simulink_extras/Transformations/Degrees to Radians
  Gain : Gain  Gain=(jointUpperLimit-jointLowerLimit)/2
  Stiffness : Gain  Gain=jointStiffness
  Sum1 : Sum  Inputs=|+-
  Sum2 : Sum  Inputs=|+-
  Torque Saturate : Saturate  UpperLimit=jointTorqueLimit  LowerLimit=-jointTorqueLimit  ZeroCross=off
  Torque : Outport
  wires:
  Damping/1 -> Sum1/2
  Stiffness/1 -> Sum1/1
  Add Constant/1 -> Degrees to Radians/1
  Gain/1 -> Add Constant/1
  Control Input/1 -> Gain/1
  Sum2/1 -> Stiffness/1
  Joint Velocity/1 -> Damping/1
  Sum1/1 -> Torque Saturate/1
  Torque Saturate/1 -> Torque/1
  Degrees to Radians/1 -> Sum2/1
  Joint Position/1 -> Sum2/2

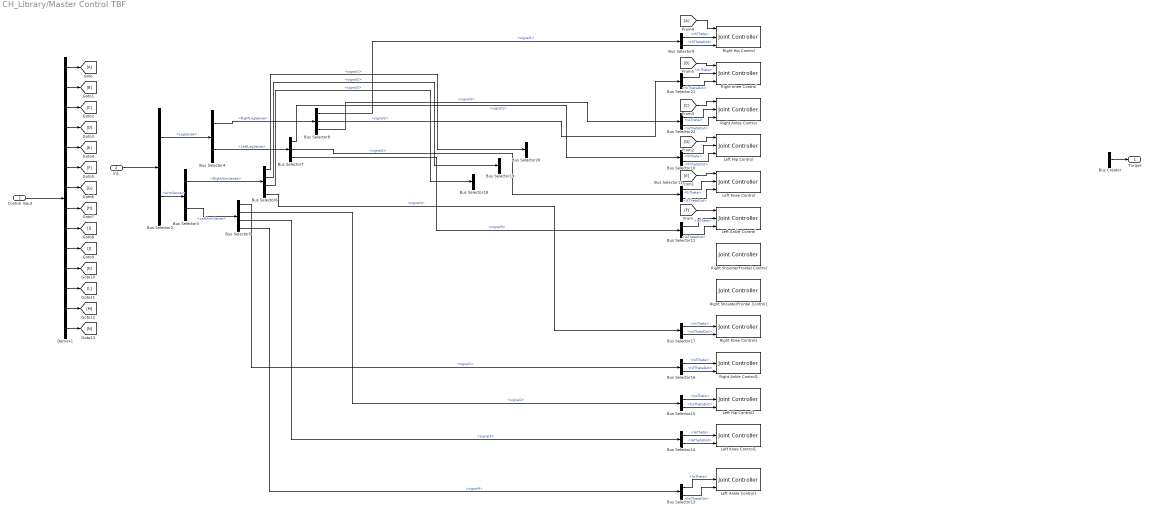
== system CH_Library/Master Control TBF ==
  Control Input : Inport
  In1 : Inport  Port=2
  Bus Creator : BusCreator  Inputs=2
  Bus Selector10 : BusSelector  OutputSignals=lhTheta,lhThetaDot
  Bus Selector11 : BusSelector  OutputSignals=lkTheta,lkThetaDot
  Bus Selector12 : BusSelector  OutputSignals=laTheta,laThetaDot
  Bus Selector13 : BusSelector  OutputSignals=lwTheta,lwThetaDot
  Bus Selector14 : BusSelector  OutputSignals=leTheta,leThetaDot
  Bus Selector15 : BusSelector  OutputSignals=lssTheta,lssThetaDot
  Bus Selector16 : BusSelector  OutputSignals=lsfTheta,lsfThetaDot
  Bus Selector17 : BusSelector  OutputSignals=rwTheta,rwThetaDot
  Bus Selector18 : BusSelector  OutputSignals=reTheta,reThetaDot
  Bus Selector19 : BusSelector  OutputSignals=rssTheta,rssThetaDot
  Bus Selector2 : BusSelector  OutputSignals=LegSense,ArmSense
  Bus Selector20 : BusSelector  OutputSignals=rsfTheta,rsfThetaDot
  Bus Selector21 : BusSelector  OutputSignals=rkTheta,rkThetaDot
  Bus Selector22 : BusSelector  OutputSignals=raTheta,raThetaDot
  Bus Selector3 : BusSelector  OutputSignals=RightArmSense,LeftArmSense
  Bus Selector4 : BusSelector  OutputSignals=RightLegSense,LeftLegSense
  Bus Selector5 : BusSelector  OutputSignals=signal1,signal2,signal3,signal4
  Bus Selector6 : BusSelector  OutputSignals=signal1,signal2,signal3,signal4
  Bus Selector7 : BusSelector  OutputSignals=signal1,signal2,signal3
  Bus Selector8 : BusSelector  OutputSignals=signal1,signal2,signal3
  Bus Selector9 : BusSelector  OutputSignals=rhTheta,rhThetaDot
  Demux1 : Demux  Outputs=14
  Left Ankle Control : sm_humanoid_walker_lib/Joint Controller  jointStiffness=params.controller.ankleStiffness  jointDamping=params.controller.ankleDamping  jointUpperLimit=params.jointLimits.ankleUpperLimit  jointLowerLimit=params.jointLimits.ankleLowerLimit  jointTorqueLimit=params.torqueLimits.ankle
  Left Ankle Control1 : sm_humanoid_walker_lib/Joint Controller  jointStiffness=params.controller.ankleStiffness  jointDamping=params.controller.ankleDamping  jointUpperLimit=params.jointLimits.ankleUpperLimit  jointLowerLimit=params.jointLimits.ankleLowerLimit  jointTorqueLimit=params.torqueLimits.ankle
  Left Hip Control : sm_humanoid_walker_lib/Joint Controller  jointStiffness=params.controller.hipFrontalStiffness  jointDamping=params.controller.hipFrontalDamping  jointUpperLimit=params.jointLimits.hipFrontalUpperLimit  jointLowerLimit=params.jointLimits.hipFrontalLowerLimit  jointTorqueLimit=params.torqueLimits.hipFrontal
  Left Hip Control1 : sm_humanoid_walker_lib/Joint Controller  jointStiffness=params.controller.hipFrontalStiffness  jointDamping=params.controller.hipFrontalDamping  jointUpperLimit=params.jointLimits.hipFrontalUpperLimit  jointLowerLimit=params.jointLimits.hipFrontalLowerLimit  jointTorqueLimit=params.torqueLimits.hipFrontal
  Left Knee Control : sm_humanoid_walker_lib/Joint Controller  jointStiffness=params.controller.kneeStiffness  jointDamping=params.controller.kneeDamping  jointUpperLimit=params.jointLimits.kneeUpperLimit  jointLowerLimit=params.jointLimits.kneeLowerLimit  jointTorqueLimit=params.torqueLimits.knee
  Left Knee Control1 : sm_humanoid_walker_lib/Joint Controller  jointStiffness=params.controller.kneeStiffness  jointDamping=params.controller.kneeDamping  jointUpperLimit=params.jointLimits.kneeUpperLimit  jointLowerLimit=params.jointLimits.kneeLowerLimit  jointTorqueLimit=params.torqueLimits.knee
  Right Ankle Control : sm_humanoid_walker_lib/Joint Controller  jointStiffness=params.controller.ankleStiffness  jointDamping=params.controller.ankleDamping  jointUpperLimit=params.jointLimits.ankleUpperLimit  jointLowerLimit=params.jointLimits.ankleLowerLimit  jointTorqueLimit=params.torqueLimits.ankle
  Right Ankle Control1 : sm_humanoid_walker_lib/Joint Controller  jointStiffness=params.controller.ankleStiffness  jointDamping=params.controller.ankleDamping  jointUpperLimit=params.jointLimits.ankleUpperLimit  jointLowerLimit=params.jointLimits.ankleLowerLimit  jointTorqueLimit=params.torqueLimits.ankle
  Right Hip Control : sm_humanoid_walker_lib/Joint Controller  jointStiffness=params.controller.hipFrontalStiffness  jointDamping=params.controller.hipFrontalDamping  jointUpperLimit=params.jointLimits.hipFrontalUpperLimit  jointLowerLimit=params.jointLimits.hipFrontalLowerLimit  jointTorqueLimit=params.torqueLimits.hipFrontal
  Right Knee Control : sm_humanoid_walker_lib/Joint Controller  jointStiffness=params.controller.kneeStiffness  jointDamping=params.controller.kneeDamping  jointUpperLimit=params.jointLimits.kneeUpperLimit  jointLowerLimit=params.jointLimits.kneeLowerLimit  jointTorqueLimit=params.torqueLimits.knee
  Right Knee Control1 : sm_humanoid_walker_lib/Joint Controller  jointStiffness=params.controller.kneeStiffness  jointDamping=params.controller.kneeDamping  jointUpperLimit=params.jointLimits.kneeUpperLimit  jointLowerLimit=params.jointLimits.kneeLowerLimit  jointTorqueLimit=params.torqueLimits.knee
  Right ShoulderFrontal Control : sm_humanoid_walker_lib/Joint Controller  jointStiffness=params.controller.hipFrontalStiffness  jointDamping=params.controller.hipFrontalDamping  jointUpperLimit=params.jointLimits.shoulderFrontalUpperLimit  jointLowerLimit=params.jointLimits.shoulderFrontalLowerLimit  jointTorqueLimit=params.torqueLimits.hipFrontal
  Right ShoulderFrontal Control1 : sm_humanoid_walker_lib/Joint Controller  jointStiffness=params.controller.hipFrontalStiffness  jointDamping=params.controller.hipFrontalDamping  jointUpperLimit=params.jointLimits.shoulderFrontalUpperLimit  jointLowerLimit=params.jointLimits.shoulderFrontalLowerLimit  jointTorqueLimit=params.torqueLimits.hipFrontal
  Torque : Outport
  wires:
  Control Input/1 -> Demux1/1
  Demux1/1 -> [A]
  Demux1/6 -> [F]
  Demux1/5 -> [E]
  Demux1/4 -> [D]
  Demux1/3 -> [C]
  Demux1/2 -> [B]
  [F] -> Left Ankle Control/1
  [E] -> Left Knee Control/1
  [D] -> Left Hip Control/1
  [C] -> Right Ankle Control/1
  [B] -> Right Knee Control/1
  Demux1/7 -> [G]
  Demux1/8 -> [H]
  Demux1/9 -> [I]
  Demux1/10 -> [J]
  Demux1/11 -> [K]
  Demux1/12 -> [L]
  Bus Creator/1 -> Torque/1
  ? -> Bus Creator/1
  Demux1/13 -> [M]
  Demux1/14 -> [N]
  Bus Selector7/2 -> Bus Selector11/1  "<signal2>"
  Bus Selector6/1 -> Bus Selector20/1  "<signal1>"
  Bus Selector4/2 -> Bus Selector7/1  "<LeftLegSense>"
  Bus Selector8/3 -> Bus Selector22/1  "<signal3>"
  Bus Selector8/1 -> Bus Selector9/1  "<signal1>"
  Bus Selector3/1 -> Bus Selector6/1  "<RightArmSense>"
  Bus Selector2/2 -> Bus Selector3/1  "<ArmSense>"
  Bus Selector7/1 -> Bus Selector10/1  "<signal1>"
  Bus Selector7/3 -> Bus Selector12/1  "<signal3>"
  In1/1 -> Bus Selector2/1
  Bus Selector8/2 -> Bus Selector21/1  "<signal2>"
  Bus Selector4/1 -> Bus Selector8/1  "<RightLegSense>"
  Bus Selector5/3 -> Bus Selector14/1  "<signal3>"
  Bus Selector6/2 -> Bus Selector19/1  "<signal2>"
  Bus Selector3/2 -> Bus Selector5/1  "<LeftArmSense>"
  Bus Selector5/4 -> Bus Selector13/1  "<signal4>"
  Bus Selector5/1 -> Bus Selector16/1  "<signal1>"
  Bus Selector6/4 -> Bus Selector17/1  "<signal4>"
  Bus Selector5/2 -> Bus Selector15/1  "<signal2>"
  Bus Selector6/3 -> Bus Selector18/1  "<signal3>"
  Bus Selector2/1 -> Bus Selector4/1  "<LegSense>"
  Bus Selector9/1 -> Right Hip Control/2  "<rhTheta>"
  Bus Selector9/2 -> Right Hip Control/3  "<rhThetaDot>"
  [A] -> Right Hip Control/1
  Bus Selector21/1 -> Right Knee Control/2  "<rkTheta>"
  Bus Selector21/2 -> Right Knee Control/3  "<rkThetaDot>"
  Bus Selector22/1 -> Right Ankle Control/2  "<raTheta>"
  Bus Selector22/2 -> Right Ankle Control/3  "<raThetaDot>"
  Bus Selector10/1 -> Left Hip Control/2  "<lhTheta>"
  Bus Selector10/2 -> Left Hip Control/3  "<lhThetaDot>"
  Bus Selector11/1 -> Left Knee Control/2  "<lkTheta>"
  Bus Selector11/2 -> Left Knee Control/3  "<lkThetaDot>"
  Bus Selector12/1 -> Left Ankle Control/2  "<laTheta>"
  Bus Selector12/2 -> Left Ankle Control/3  "<laThetaDot>"
  Bus Selector13/2 -> Left Ankle Control1/3  "<lwThetaDot>"
  Bus Selector13/1 -> Left Ankle Control1/2  "<lwTheta>"
  Bus Selector14/1 -> Left Knee Control1/2  "<leTheta>"
  Bus Selector14/2 -> Left Knee Control1/3  "<leThetaDot>"
  Bus Selector15/2 -> Left Hip Control1/3  "<lssThetaDot>"
  Bus Selector15/1 -> Left Hip Control1/2  "<lssTheta>"
  Bus Selector16/1 -> Right Ankle Control1/2  "<lsfTheta>"
  Bus Selector16/2 -> Right Ankle Control1/3  "<lsfThetaDot>"
  Bus Selector17/2 -> Right Knee Control1/3  "<rwThetaDot>"
  Bus Selector17/1 -> Right Knee Control1/2  "<rwTheta>"

== system CH_Library/Obj to corner Collisions ==
  Simscape Bus : SimscapeBus  HierarchyStrings=Connection1;Connection2;Connection3;Connection4;Connection5;Connection6;Connection7;Connection8
  Spatial Contact Force{,1..7} (8 alike) : sm_lib/Forces and Torques/Spatial Contact Force  CoefficientOfDynamicFriction=MatDynFric  CoefficientOfStaticFriction=MatStatFric  SenseContactBaseRotation=off  SenseContactBaseTranslation=off  NormalDamping=MatDamp  NormalDampingUnits=N/(m/s)  SenseContactFollowerRotation=off  SenseContactFollowerTranslation=off  SenseContactSignal=off  NormalStiffness=MatStiff  NormalStiffnessUnits=N/m  FrictionalCriticalVelocity=CritVel  FrictionalCriticalVelocityUnits=m/s  ZeroCrossDetectContactStartAndEnd=off  FrictionType=SmoothStickSlip  SenseFrictionalForceMagnitude=off  SenseNormalForceMagnitude=off  NormalForceType=SmoothSpringDamper  SenseNormalVelocity=off  SenseSeparationDistance=off  SenseTangentialVelocity=off  SenseTangentialVelocityMagnitude=off  NormalTransitionRegionWidth=TransitionRegion  NormalTransitionRegionWidthUnits=m
  Single Object : PMIOPort  Side=Right
  Box : PMIOPort  Port=2  Side=Left
  connections:
  Spatial Contact Force/LConn1 -- Simscape Bus/LConn1
  Spatial Contact Force1/LConn1 -- Simscape Bus/LConn2
  Spatial Contact Force2/LConn1 -- Simscape Bus/LConn3
  Spatial Contact Force3/LConn1 -- Simscape Bus/LConn4
  Spatial Contact Force4/LConn1 -- Simscape Bus/LConn5
  Spatial Contact Force5/LConn1 -- Simscape Bus/LConn6
  Spatial Contact Force6/LConn1 -- Simscape Bus/LConn7
  Single Object/RConn1 -- Spatial Contact Force/RConn1 -- Spatial Contact Force1/RConn1 -- Spatial Contact Force2/RConn1 -- Spatial Contact Force3/RConn1 -- Spatial Contact Force5/RConn1 -- Spatial Contact Force6/RConn1 -- Spatial Contact Force7/RConn1 -- Spatial Contact Force4/RConn1
  Box/RConn1 -- Simscape Bus/RConn1
  Spatial Contact Force7/LConn1 -- Simscape Bus/LConn8

== system CH_Library/Real Actuator ==
  Voltage : Inport
  Controlled Voltage Source : fl_lib/Electrical/Electrical Sources/Controlled Voltage Source
  DC Motor : ee_lib/Electromechanical/Brushed Motors/DC Motor  field_option=ee.enum.field_option.pm  Rf=100 Ohm  Lf=1 H  Laf=0.15 H  If0=0 A  parameterization=ee.enum.dcparam_option.torque_speed  Ra=3.9 Ohm  La=ArmatureInductance H  emf_or_torque=ee.enum.emf_or_torque.ki  Kv=0.072e-3 V/rpm  Ki=6.876e-4 N*m/A  T_stall=StallTorque N*m  w_max="NoLoadSpeed   rpm"  w_rated=15000 rpm  P_rated=0.08 W  V_rated=RatedDCSupply V  J=0.01 g*cm^2  lam_param=ee.enum.lam_param.damping  lam=0 N*m/(rad/s)  i_noload=0 A  V_i_noload=1.5 V  speed0=0 rpm  enable_fault_armature=ee.enum.faults.faultEnable.no  rev_faulted=1 / 3  G_faulted_armature=1e-5 S  fault_trigger_armature=ee.enum.faults.faultTrigger.behavioral  t_fault_armature=1 s  max_permissible_current_armature=4 A  t_fail_on_current_armature=1 s  enable_fault_field=ee.enum.faults.faultEnable.no  G_faulted_field=1e-5 S  fault_trigger_field=ee.enum.faults.faultTrigger.temporal  t_fault_field=1 s  max_permissible_current_field=inf A  t_fail_on_current_field=1 s  fault_action=ee.enum.faults.faultAction.none  alpha=3.93e-3 1/K  Tmeas=25 degC  thermal_mass=100 J/K  initial_temperature=25 degC
  Electrical Reference : fl_lib/Electrical/Electrical Elements/Electrical Reference
  Mechanical Rotational Reference : fl_lib/Mechanical/Rotational Elements/Mechanical Rotational Reference
  Rotational Multibody Interface1 : fl_lib/Mechanical/Multibody Interfaces/Rotational Multibody Interface
      settings: SourceProductBaseCode=SS
  Simulink-PS Converter : nesl_utility/Simulink-PS Converter  PhysicalDomain=network_engine_domain  SubClassName=ps_input  LeftPortType=input  RightPortType=output  PseudoPeriodic=off  Frequencies=[]  NoiseDistribution=none  NoiseParameters=[]  Unit=1  AffineConversion=off  FilteringAndDerivatives=provide  SimscapeFilterOrder=1  InputFilterTimeConstant=0.001  UdotUserProvided=0
      settings: SourceProductBaseCode=PW,SS
  T : PMIOPort  Side=Left
  W : PMIOPort  Port=2  Side=Left
  wires:
  Voltage/1 -> Simulink-PS Converter/1
  connections:
  Rotational Multibody Interface1/RConn1 -- W/RConn1
  Rotational Multibody Interface1/LConn1 -- T/RConn1
  Simulink-PS Converter/RConn1 -- Controlled Voltage Source/RConn1
  Controlled Voltage Source/RConn2 -- DC Motor/LConn1
  Controlled Voltage Source/LConn1 -- DC Motor/RConn1 -- Electrical Reference/LConn1
  DC Motor/LConn2 -- Rotational Multibody Interface1/LConn2
  DC Motor/RConn2 -- Rotational Multibody Interface1/RConn2 -- Mechanical Rotational Reference/LConn1
